simulink model "sl_subsys_iferr1"  (Simulink 6.0)
settings: Solver=FixedStepDiscrete  StartTime=0.0  StopTime=10.0  FixedStep=1  RelTol=1e-3
settings Model: CovMetricSettings=d  Creator=The MathWorks Inc.  LastModifiedBy=batserve  ExtModeAutoUpdateStatusClock=off
settings OptimizationCC: BlockReduction=off  BooleanDataType=off
settings DebuggingCC: CheckExecutionContextPreStartOutputMsg=on  CheckExecutionContextRuntimeOutputMsg=on  SolverPrmCheckMsg=none
settings HardwareCC: TargetUnknown=on

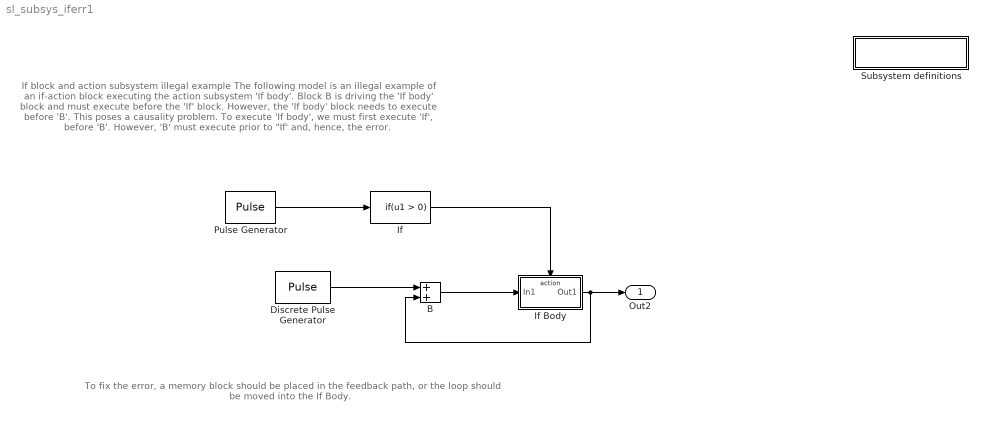
== system sl_subsys_iferr1 ==
  note: If block and action subsystem illegal example
      |
      | The following model is an illegal example of an if-action block executing the
      | action subsystem 'If body'. Block B is driving the 'If body' block and
      | must execute before the 'If' block. However, the 'If body' block needs to execute
      | before 'B'. This poses a causality problem.  To execute 'If body', we must
      | first execute 'If', before 'B'. However, 'B' must execute prior to
      | "If' and, hence, the error.
  note: To fix the error, a memory block should be placed in the feedback path, or
      | the loop should be moved into the If Body.
  " Subsystem definitions" : Subsystem  PropExecContextAcrossSSBoundary=on
      settings: OpenFcn=helpview([matlabroot,'/toolbox/simulink/simdemos/sl_subsys_definitions.html']);
      mask Display: disp('Subsystem\ndefinitions')
  B : Sum  SaturateOnIntegerOverflow=on  InputSameDT=on
  Discrete Pulse Generator : DiscretePulseGenerator
  If : If  ShowElse=off
  If Body : Subsystem  TreatAsAtomicUnit=on  PropExecContextAcrossSSBoundary=on
  Pulse Generator : DiscretePulseGenerator
  Out2 : Outport
  wires:
  If/1 -> If Body/Action
  Pulse Generator/1 -> If/1
  Discrete Pulse Generator/1 -> B/1
  If Body/1(Out1) -> Out2/1, B/2
  B/1 -> If Body/1(In1)

== system sl_subsys_iferr1/ Subsystem definitions ==

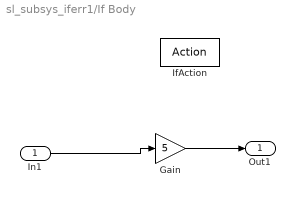
== system sl_subsys_iferr1/If Body ==
  In1 : Inport  Port=1  LatchInput=off
  IfAction : ActionPort  ActionType=then
  Gain : Gain  Gain=5  SaturateOnIntegerOverflow=on
  Out1 : Outport
  wires:
  In1/1 -> Gain/1
  Gain/1 -> Out1/1
